simulink model "BLDC_full_sysid_sim"  (R2024b)
settings: Solver=ode4  StartTime=0.0  StopTime=10.0  FixedStep=0.0001  RelTol=1e-3
values from neighbouring files (symbols this model uses):
  d = 0.35757    [DRBA_motor_EKF.m]    (also in DRBA_motor_PID_control.m; DRBA_motor_sysid.m = 0.1)
  f = 0.53378    [DRBA_motor_EKF.m]    (also in DRBA_motor_PID_control.m; DRBA_motor_sysid.m = 0.05)
  J = 0.05    [DRBA_motor_EKF.m]    (also in DRBA_motor_PID_control.m; DRBA_motor_sysid.m = 0.03)
  Kb = 20.91    [DRBA_motor_EKF.m]    (also in DRBA_motor_PID_control.m; DRBA_motor_sysid.m = 22)
  Kt = 0.7    [DRBA_motor_EKF.m]    (also in DRBA_motor_PID_control.m; DRBA_motor_sysid.m = 0.72)
  L = 0.00069    [DRBA_motor_EKF.m]    (also in DRBA_motor_PID_control.m; DRBA_motor_sysid.m = 0.00067)
  R = 0.0755    [DRBA_motor_EKF.m]    (also in DRBA_motor_PID_control.m; DRBA_motor_sysid.m = 0.0725)
settings Model: Creator=User  LastModifiedBy=User

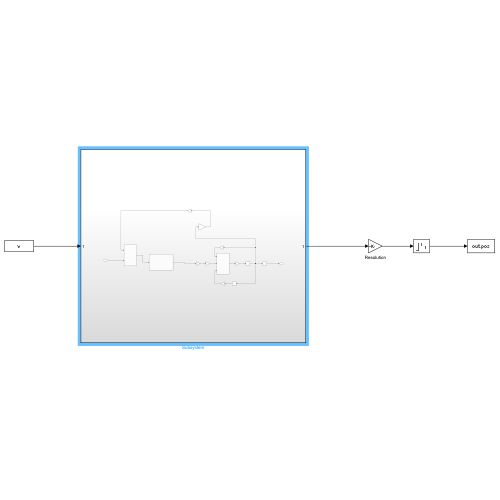
[thumbnail: Simulink's stored preview of the top-level diagram]
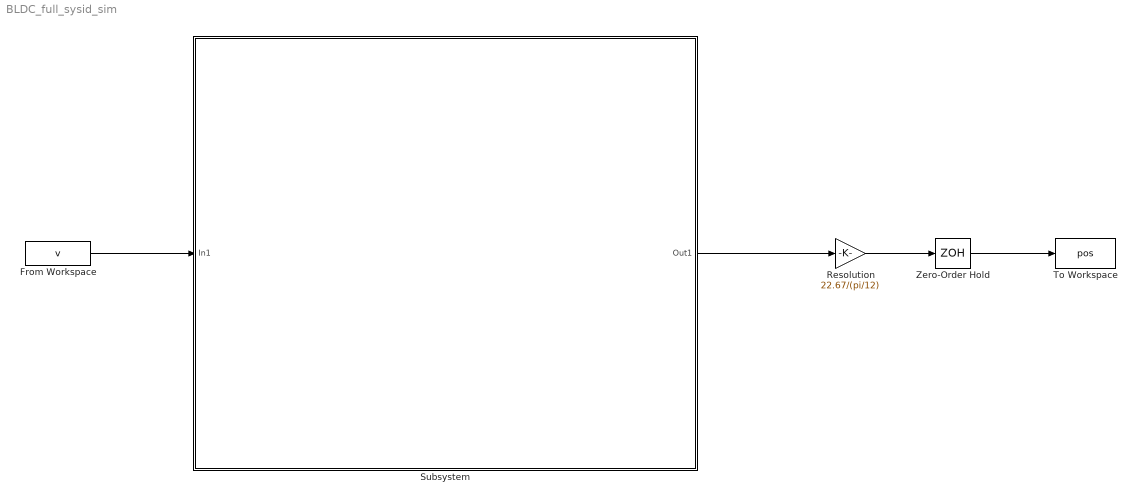
== system BLDC_full_sysid_sim ==
  From Workspace : FromWorkspace  VariableName=v
  Resolution : Gain  Gain=22.67/(pi/12)  OutDataTypeStr=int32  RndMeth=Zero  SaturateOnIntegerOverflow=on
  Subsystem : Subsystem  SystemSampleTime=0.0001
  To Workspace : ToWorkspace  VariableName=pos  SampleTime=-1
  Zero-Order Hold : ZeroOrderHold  SampleTime=0.005
  wires:
  Resolution/1 -> Zero-Order Hold/1
  From Workspace/1 -> Subsystem/1(In1)
  Subsystem/1(Out1) -> Resolution/1
  Zero-Order Hold/1 -> To Workspace/1

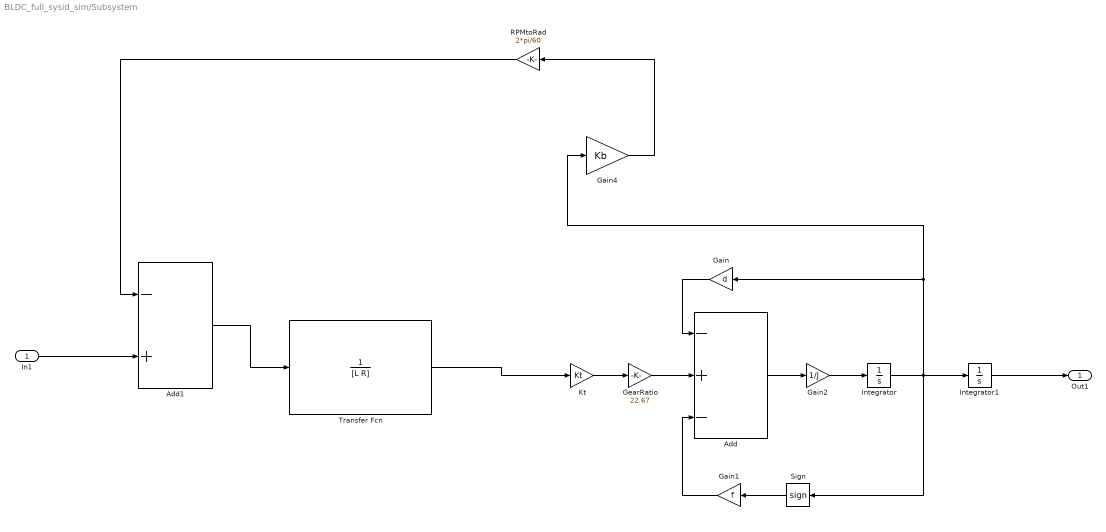
== system BLDC_full_sysid_sim/Subsystem ==
  In1 : Inport
  Add : Sum  Inputs=-+-
  Add1 : Sum  Inputs=-+
  Gain : Gain  Gain=d
  Gain1 : Gain  Gain=f
  Gain2 : Gain  Gain=1/J
  Gain4 : Gain  Gain=Kb
  GearRatio : Gain  Gain=22.67
  Integrator : Integrator
  Integrator1 : Integrator
  Kt : Gain  Gain=Kt
  RPMtoRad : Gain  Gain=2*pi/60
  Sign : Signum  ZeroCross=off
  Transfer Fcn : TransferFcn  Denominator=[L R]
  Out1 : Outport
  wires:
  Gain/1 -> Add/1
  Integrator1/1 -> Out1/1
  Kt/1 -> GearRatio/1
  GearRatio/1 -> Add/2
  RPMtoRad/1 -> Add1/1
  In1/1 -> Add1/2
  Gain2/1 -> Integrator/1
  Transfer Fcn/1 -> Kt/1
  Integrator/1 -> Integrator1/1, Gain4/1, Gain/1, Sign/1
  Add/1 -> Gain2/1
  Add1/1 -> Transfer Fcn/1
  Gain1/1 -> Add/3
  Sign/1 -> Gain1/1
  Gain4/1 -> RPMtoRad/1
